simulink model "pha_0_7_signal_logic"  (R2023a)
settings: Solver=VariableStepAuto  StartTime=0.0  StopTime=5  RelTol=1e-3
settings Model: PacingRate=0.500000  Creator=Dovlica  LastModifiedBy=Dovlica
settings SimscapeCC: SimscapeLogType=all

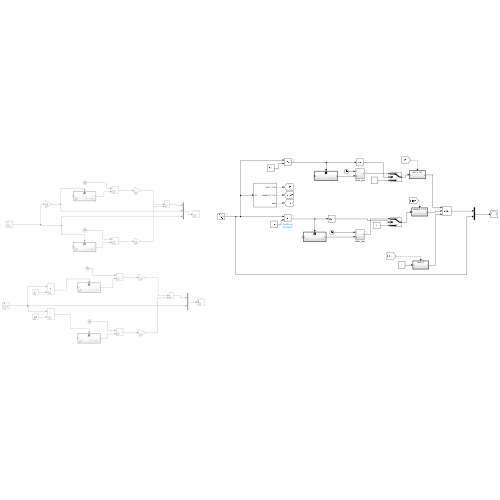
[thumbnail: Simulink's stored preview of the top-level diagram]
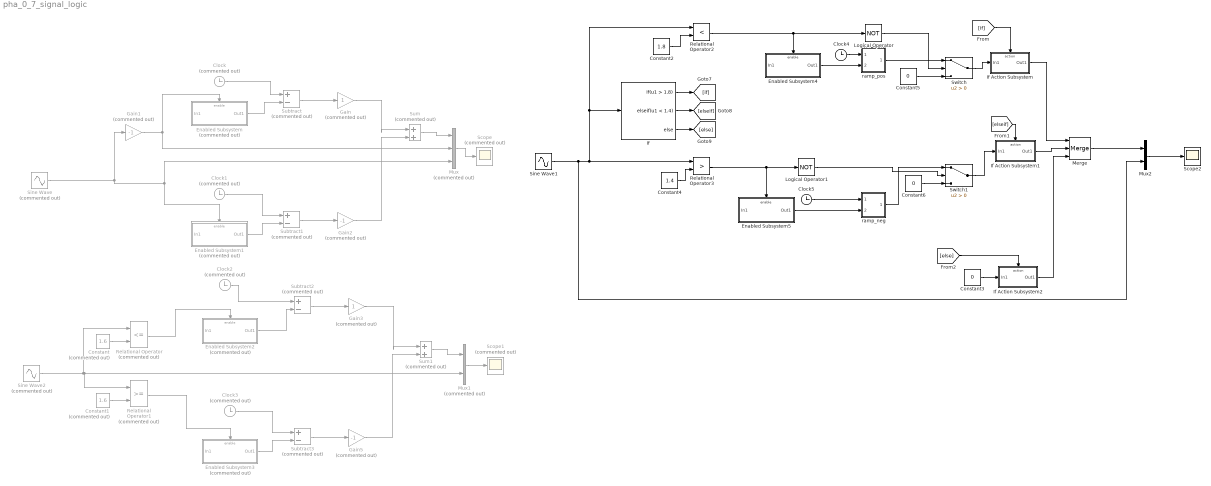
== system pha_0_7_signal_logic ==
  Clock{,1..3} (4 alike) : Clock  Commented=on
  Clock4 : Clock
  Clock5 : Clock
  Constant : Constant  Commented=on  Value=1.6
  Constant1 : Constant  Commented=on  Value=1.6
  Constant2 : Constant  Value=1.8
  Constant3 : Constant  Value=0
  Constant4 : Constant  Value=1.4
  Constant5 : Constant  Value=0
  Constant6 : Constant  Value=0
  Enabled Subsystem : Subsystem  Commented=on  TreatAsAtomicUnit=on
  Enabled Subsystem1 : Subsystem  Commented=on  TreatAsAtomicUnit=on
  Enabled Subsystem2 : Subsystem  Commented=on  TreatAsAtomicUnit=on
  Enabled Subsystem3 : Subsystem  Commented=on  TreatAsAtomicUnit=on
  Enabled Subsystem4 : Subsystem  TreatAsAtomicUnit=on
  Enabled Subsystem5 : Subsystem  TreatAsAtomicUnit=on
  Gain : Gain  Commented=on
  Gain1 : Gain  Commented=on  Gain=-1
  Gain2 : Gain  Commented=on  Gain=-1
  Gain3 : Gain  Commented=on
  Gain5 : Gain  Commented=on  Gain=-1
  If : If  IfExpression=u1 > 1.8  ElseIfExpressions=u1 < 1.4
  If Action Subsystem : Subsystem  TreatAsAtomicUnit=on
  If Action Subsystem1 : Subsystem  TreatAsAtomicUnit=on
  If Action Subsystem2 : Subsystem  TreatAsAtomicUnit=on
  Logical Operator : Logic  Operator=NOT  AllPortsSameDT=off  OutDataTypeStr=boolean
  Logical Operator1 : Logic  Operator=NOT  AllPortsSameDT=off  OutDataTypeStr=boolean
  Merge : Merge  Inputs=3
  Mux : Mux  Commented=on  Inputs=3
  Mux1 : Mux  Commented=on  Inputs=2
  Mux2 : Mux  Inputs=2
  Relational Operator : RelationalOperator  Commented=on  Operator=<=  OutDataTypeStr=boolean  RndMeth=Simplest  InputSameDT=off
  Relational Operator1 : RelationalOperator  Commented=on  OutDataTypeStr=boolean  RndMeth=Simplest  InputSameDT=off
  Relational Operator2 : RelationalOperator  Operator=<  OutDataTypeStr=boolean  RndMeth=Simplest  InputSameDT=off
  Relational Operator3 : RelationalOperator  Operator=>  OutDataTypeStr=boolean  RndMeth=Simplest  InputSameDT=off
  Scope : Scope  Commented=on
  Scope1 : Scope  Commented=on
  Scope2 : Scope
  Sine Wave : Sin  Commented=on  Amplitude=0.21  Bias=1.6  SampleTime=0
  Sine Wave1 : Sin  Amplitude=0.21  Bias=1.6  Frequency=5  SampleTime=0
  Sine Wave2 : Sin  Commented=on  Amplitude=0.21  Bias=1.6  SampleTime=0
  Subtract{,1..3} (4 alike) : Sum  Commented=on  Inputs=+-
  Sum : Sum  Commented=on  Inputs=|++
  Sum1 : Sum  Commented=on  Inputs=|++
  Switch : Switch  Criteria=u2 > Threshold  SaturateOnIntegerOverflow=off  InputSameDT=off
  Switch1 : Switch  Criteria=u2 > Threshold  SaturateOnIntegerOverflow=off  InputSameDT=off
  ramp_neg : Subsystem
  ramp_pos : Subsystem
  wires:
  Clock/1 -> Subtract/1
  Enabled Subsystem/1(Out1) -> Subtract/2
  Sine Wave/1 -> Mux/3, Enabled Subsystem1/Enable, Gain1/1
  Subtract/1 -> Gain/1
  Gain/1 -> Sum/1
  Mux/1 -> Scope/1
  Gain1/1 -> Enabled Subsystem/Enable, Mux/2
  Enabled Subsystem1/1(Out1) -> Subtract1/2
  Clock1/1 -> Subtract1/1
  Subtract1/1 -> Gain2/1
  Gain2/1 -> Sum/2
  Sum/1 -> Mux/1
  If/1 -> [if]
  If/2 -> [elseif]
  If/3 -> [else]
  Sine Wave1/1 -> If/1, Relational Operator2/1, Relational Operator3/1, Mux2/2
  Sine Wave2/1 -> Relational Operator1/1, Mux1/2, Relational Operator/1
  Sum1/1 -> Mux1/1
  Gain5/1 -> Sum1/2
  Enabled Subsystem3/1(Out1) -> Subtract3/2
  Clock3/1 -> Subtract3/1
  Subtract3/1 -> Gain5/1
  Subtract2/1 -> Gain3/1
  Mux1/1 -> Scope1/1
  Clock2/1 -> Subtract2/1
  Enabled Subsystem2/1(Out1) -> Subtract2/2
  Gain3/1 -> Sum1/1
  Constant/1 -> Relational Operator/2
  Relational Operator/1 -> Enabled Subsystem2/Enable
  Constant1/1 -> Relational Operator1/2
  Relational Operator1/1 -> Enabled Subsystem3/Enable
  [if] -> If Action Subsystem/Action
  [elseif] -> If Action Subsystem1/Action
  [else] -> If Action Subsystem2/Action
  Mux2/1 -> Scope2/1
  Merge/1 -> Mux2/1
  If Action Subsystem1/1(Out1) -> Merge/2
  Enabled Subsystem4/1(Out1) -> ramp_pos/2(In2)
  Clock4/1 -> ramp_pos/1(In1)
  Constant2/1 -> Relational Operator2/2
  Relational Operator2/1 -> Logical Operator/1, Enabled Subsystem4/Enable
  ramp_pos/1(Out1) -> Switch/1
  If Action Subsystem/1(Out1) -> Merge/1
  Constant4/1 -> Relational Operator3/2
  Enabled Subsystem5/1(Out1) -> ramp_neg/2(In2)
  Clock5/1 -> ramp_neg/1(In1)
  If Action Subsystem2/1(Out1) -> Merge/3
  Relational Operator3/1 -> Logical Operator1/1, Enabled Subsystem5/Enable
  Constant3/1 -> If Action Subsystem2/1(In1)
  Logical Operator/1 -> Switch/2
  Constant5/1 -> Switch/3
  Logical Operator1/1 -> Switch1/2
  ramp_neg/1(Out1) -> Switch1/1
  Constant6/1 -> Switch1/3
  Switch1/1 -> If Action Subsystem1/1(In1)
  Switch/1 -> If Action Subsystem/1(In1)

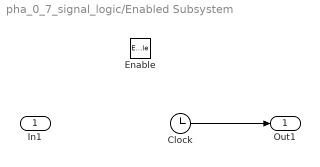
== system pha_0_7_signal_logic/Enabled Subsystem ==
  In1 : Inport
  Enable : EnablePort
  Clock : Clock
  Out1 : Outport
  wires:
  Clock/1 -> Out1/1

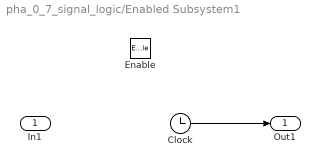
== system pha_0_7_signal_logic/Enabled Subsystem1 ==
  In1 : Inport
  Enable : EnablePort
  Clock : Clock
  Out1 : Outport
  wires:
  Clock/1 -> Out1/1

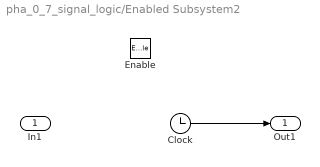
== system pha_0_7_signal_logic/Enabled Subsystem2 ==
  In1 : Inport
  Enable : EnablePort
  Clock : Clock
  Out1 : Outport
  wires:
  Clock/1 -> Out1/1

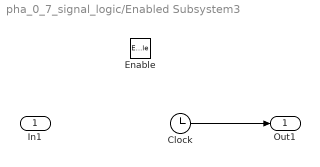
== system pha_0_7_signal_logic/Enabled Subsystem3 ==
  In1 : Inport
  Enable : EnablePort
  Clock : Clock
  Out1 : Outport
  wires:
  Clock/1 -> Out1/1

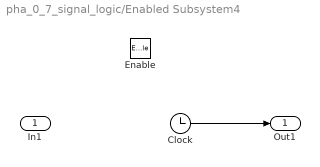
== system pha_0_7_signal_logic/Enabled Subsystem4 ==
  In1 : Inport
  Enable : EnablePort
  Clock : Clock
  Out1 : Outport
  wires:
  Clock/1 -> Out1/1

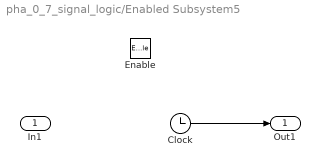
== system pha_0_7_signal_logic/Enabled Subsystem5 ==
  In1 : Inport
  Enable : EnablePort
  Clock : Clock
  Out1 : Outport
  wires:
  Clock/1 -> Out1/1

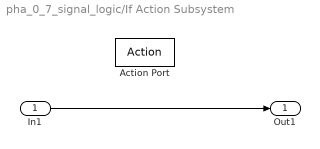
== system pha_0_7_signal_logic/If Action Subsystem ==
  In1 : Inport
  Action Port : ActionPort  ActionPortLabel=if(u1 > 1.8)
  Out1 : Outport
  wires:
  In1/1 -> Out1/1

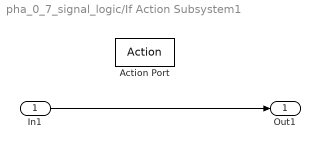
== system pha_0_7_signal_logic/If Action Subsystem1 ==
  In1 : Inport
  Action Port : ActionPort  ActionPortLabel=elseif(u1 < 1.4)
  Out1 : Outport
  wires:
  In1/1 -> Out1/1

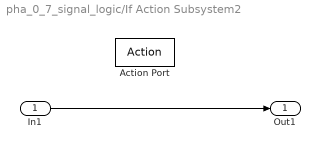
== system pha_0_7_signal_logic/If Action Subsystem2 ==
  In1 : Inport
  Action Port : ActionPort  ActionPortLabel=else
  Out1 : Outport
  wires:
  In1/1 -> Out1/1

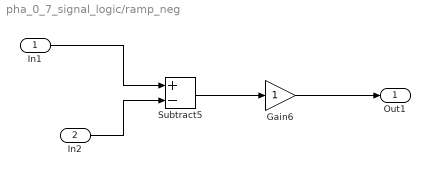
== system pha_0_7_signal_logic/ramp_neg ==
  In1 : Inport
  In2 : Inport  Port=2
  Gain6 : Gain
  Subtract5 : Sum  Inputs=+-
  Out1 : Outport
  wires:
  Subtract5/1 -> Gain6/1
  In1/1 -> Subtract5/1
  Gain6/1 -> Out1/1
  In2/1 -> Subtract5/2

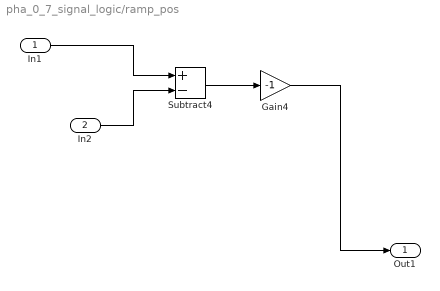
== system pha_0_7_signal_logic/ramp_pos ==
  In1 : Inport
  In2 : Inport  Port=2
  Gain4 : Gain  Gain=-1
  Subtract4 : Sum  Inputs=+-
  Out1 : Outport
  wires:
  Subtract4/1 -> Gain4/1
  Gain4/1 -> Out1/1
  In1/1 -> Subtract4/1
  In2/1 -> Subtract4/2
